simulink model "identificacaoPlanta"  (R2015a)
settings: Solver=ode1  StartTime=0.0  StopTime=8  FixedStep=0.0321  RelTol=1e-3
values from neighbouring files (symbols this model uses):
  gainAtuador = 5/255*0.05/0.0475*2    (= 0.0412796697626)    [identificacaoRobot.m]    (also in scriptIdentificacaoDoRobo.m)
  refTheta = robotData(:,5)*180/pi    [identificacaoRobot.m]
  theta = robotData(:,6)*180/pi    [identificacaoRobot.m]
  ur = v1-v2    [identificacaoRobot.m]
  v1 = sinalTensao1*5/255    [identificacaoRobot.m]
settings Model: Creator=Jean  LastModifiedBy=jean-lucas

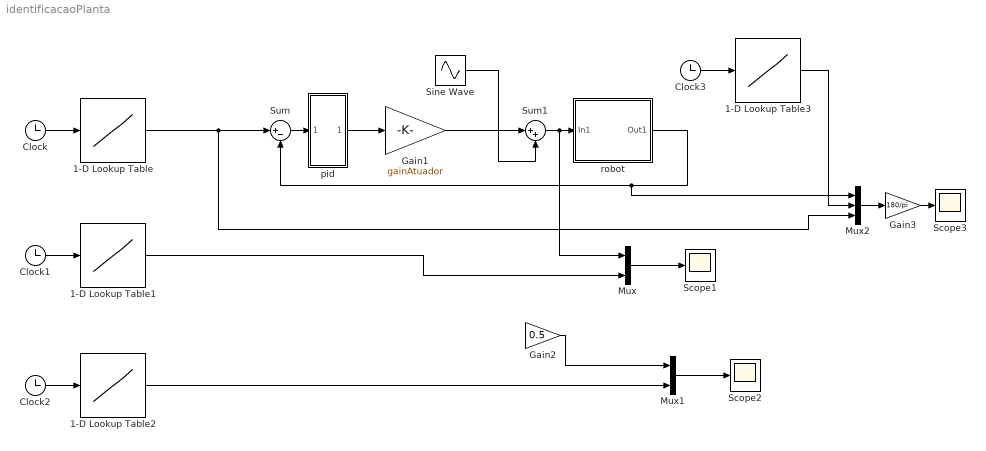
== system identificacaoPlanta ==
  1-D Lookup Table : Lookup_n-D  NumberOfTableDimensions=1  BreakpointsForDimension1=t  Table=refTheta*pi/180  InternalRulePriority=Speed  RndMeth=Simplest  InputSameDT=on
  1-D Lookup Table1 : Lookup_n-D  NumberOfTableDimensions=1  BreakpointsForDimension1=t  Table=ur  InternalRulePriority=Speed  RndMeth=Simplest  InputSameDT=on
  1-D Lookup Table2 : Lookup_n-D  NumberOfTableDimensions=1  BreakpointsForDimension1=t  Table=v1  InternalRulePriority=Speed  RndMeth=Simplest  InputSameDT=on
  1-D Lookup Table3 : Lookup_n-D  NumberOfTableDimensions=1  BreakpointsForDimension1=t  Table=theta*pi/180  InternalRulePriority=Speed  RndMeth=Simplest  InputSameDT=on
  Clock{,1..3} (4 alike) : Clock
  Gain1 : Gain  Gain=gainAtuador
  Gain2 : Gain  Gain=0.5
  Gain3 : Gain  Gain=180/pi
  Mux : Mux  Inputs=2
  Mux1 : Mux  Inputs=2
  Mux2 : Mux  Inputs=3
  Scope1 : Scope
      settings: SaveName=teste
  Scope2 : Scope
      settings: SaveName=teste1
  Scope3 : Scope
      settings: SaveName=teste2
  Sine Wave : Sin  Amplitude=0.5  Frequency=2*pi*20  SampleTime=0
  Sum : Sum  Inputs=|+-
  Sum1 : Sum  Inputs=|++
  pid : Subsystem
  robot : Subsystem
  wires:
  pid/1(Out1) -> Gain1/1
  Sum/1 -> pid/1(In1)
  Gain1/1 -> Sum1/1
  robot/1(Out1) -> Mux2/1, Sum/2
  Clock/1 -> 1-D Lookup Table/1
  1-D Lookup Table/1 -> Mux2/3, Sum/1
  Clock1/1 -> 1-D Lookup Table1/1
  1-D Lookup Table1/1 -> Mux/2
  Mux/1 -> Scope1/1
  Gain2/1 -> Mux1/1
  1-D Lookup Table2/1 -> Mux1/2
  Mux1/1 -> Scope2/1
  Clock2/1 -> 1-D Lookup Table2/1
  Clock3/1 -> 1-D Lookup Table3/1
  Mux2/1 -> Gain3/1
  Gain3/1 -> Scope3/1
  1-D Lookup Table3/1 -> Mux2/2
  Sum1/1 -> Mux/1, robot/1(In1)
  Sine Wave/1 -> Sum1/2

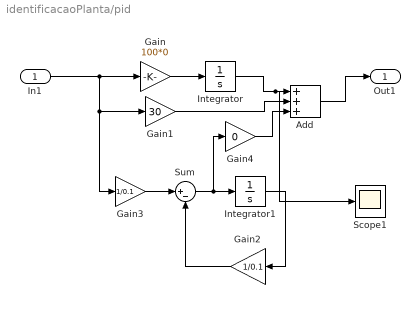
== system identificacaoPlanta/pid ==
  In1 : Inport
  Add : Sum  Inputs=+++
  Gain : Gain  Gain=100*0
  Gain1 : Gain  Gain=30
  Gain2 : Gain  Gain=1/0.1
  Gain3 : Gain  Gain=1/0.1
  Gain4 : Gain  Gain=0
  Integrator : Integrator
  Integrator1 : Integrator
  Scope1 : Scope
      settings: SaveName=teste4
  Sum : Sum  Inputs=|+-
  Out1 : Outport
  wires:
  Gain/1 -> Integrator/1
  In1/1 -> Gain3/1, Gain1/1, Gain/1
  Add/1 -> Out1/1
  Integrator/1 -> Scope1/1, Add/1
  Gain1/1 -> Add/2
  Sum/1 -> Gain4/1, Integrator1/1
  Integrator1/1 -> Gain2/1
  Gain2/1 -> Sum/2
  Gain3/1 -> Sum/1
  Gain4/1 -> Add/3

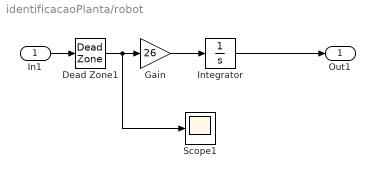
== system identificacaoPlanta/robot ==
  In1 : Inport
  Dead Zone1 : DeadZone  LowerValue=-0.6  UpperValue=0.6  SaturateOnIntegerOverflow=on
  Gain : Gain  Gain=26
  Integrator : Integrator  InitialCondition=36.25*pi/180
  Scope1 : Scope
      settings: SaveName=teste3
  Out1 : Outport
  wires:
  Gain/1 -> Integrator/1
  Integrator/1 -> Out1/1
  In1/1 -> Dead Zone1/1
  Dead Zone1/1 -> Scope1/1, Gain/1
